simulink model "proj2Ex"  (R2017b)
settings: Solver=VariableStepAuto  StartTime=0.0  StopTime=inf  RelTol=1e-3
libraries: libraryProject2 x4, realtime_pacer_lib x1
settings Model: Creator=BRAHIMA FANNY  LastModifiedBy=wafflefries
settings CodeAppCC: StateflowObjectComments=on

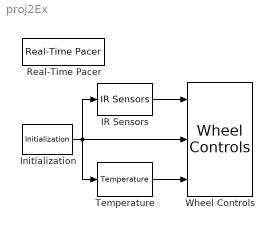
== system proj2Ex ==
  "IR Sensors " : libraryProject2/IR Sensors 
  Initialization : libraryProject2/Initialization
  Real-Time Pacer : realtime_pacer_lib/Real-Time Pacer  simTimePerRealTime=0.5
  Temperature : libraryProject2/Temperature
  Wheel Controls : libraryProject2/Wheel Controls
  wires:
  "IR Sensors "/1 -> Wheel Controls/1
  Temperature/1 -> Wheel Controls/3
  Initialization/1 -> Temperature/1, Wheel Controls/2, "IR Sensors "/1
